simulink model "move_to_ball"  (R2020a)
settings: Solver=FixedStepDiscrete  StartTime=0.0  StopTime=inf  RelTol=1e-3
model workspace (MAT data in the model file):
  SL_ROS_VariableLengthArrays_MaxSizes.CommonInfo.ArrayTruncateAction = 'EmitWarning'
  SL_ROS_VariableLengthArrays_MaxSizes.MsgTypeMap = containers.Map
  SL_ROS_VariableLengthArrays_MaxSizes.MsgTypeMap.serialization.keys = {'sensor_msgs/Image'}
  SL_ROS_VariableLengthArrays_MaxSizes.MsgTypeMap.serialization.values{1}(1).PropertyName = 'Data'
  SL_ROS_VariableLengthArrays_MaxSizes.MsgTypeMap.serialization.values{1}(1).DataType = 'uint8'
  SL_ROS_VariableLengthArrays_MaxSizes.MsgTypeMap.serialization.values{1}(1).MaxLength = 3121200
  SL_ROS_VariableLengthArrays_MaxSizes.MsgTypeMap.serialization.values{1}(2).PropertyName = 'Encoding'
  SL_ROS_VariableLengthArrays_MaxSizes.MsgTypeMap.serialization.values{1}(2).DataType = 'uint8'
  SL_ROS_VariableLengthArrays_MaxSizes.MsgTypeMap.serialization.values{1}(2).MaxLength = 128
  SL_ROS_VariableLengthArrays_MaxSizes.MsgTypeMap.serialization.uniformity = 0
  SL_ROS_VariableLengthArrays_MaxSizes.MsgTypeMap.serialization.keyType = 'char'
  SL_ROS_VariableLengthArrays_MaxSizes.MsgTypeMap.serialization.valueType = 'any'
undefined symbols (not defined in the file): gray
libraries: robotlib x8
settings Model: Creator=shiva  LastModifiedBy=shiva
settings OptimizationCC: ZeroExternalMemoryAtStartup=off  ZeroInternalMemoryAtStartup=off
settings RTWCC: TargetLang=C++
settings GRTTargetCC: TargetLangStandard=C++03 (ISO)  MultiInstanceERTCode=on  CodeInterfacePackaging=C++ class

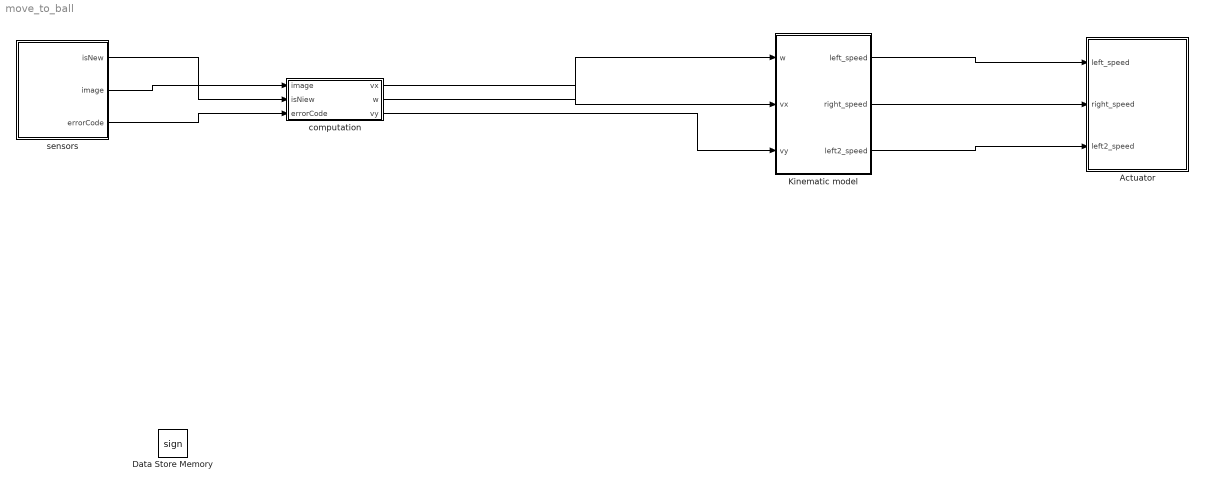
== system move_to_ball ==
  Actuator : Subsystem
  Data Store Memory : DataStoreMemory  DataStoreName=sign  ReadBeforeWriteMsg=warning  WriteAfterWriteMsg=warning  WriteAfterReadMsg=warning  ShowAdditionalParam=off
  Kinematic model : Subsystem
  computation : Subsystem
  sensors : Subsystem
  wires:
  Kinematic model/2(right_speed) -> Actuator/2(right_speed)
  Kinematic model/3(left2_speed) -> Actuator/3(left2_speed)
  Kinematic model/1(left_speed) -> Actuator/1(left_speed)
  sensors/1(isNew) -> computation/2(isNiew)
  sensors/2(image) -> computation/1(image)
  sensors/3(errorCode) -> computation/3(errorCode)
  computation/1(vx) -> Kinematic model/2(vx)
  computation/2(w) -> Kinematic model/1(w)
  computation/3(vy) -> Kinematic model/3(vy)

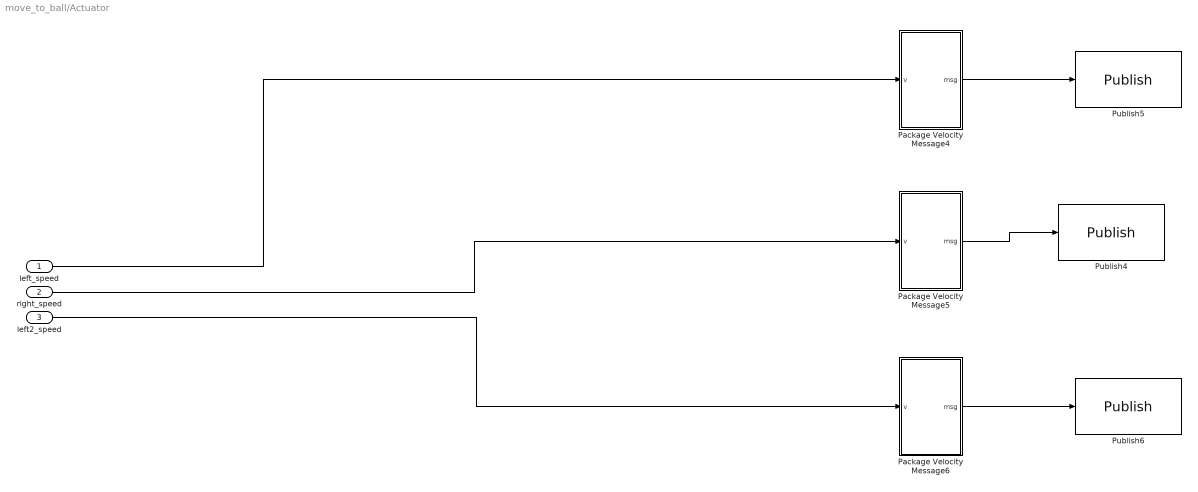
== system move_to_ball/Actuator ==
  left_speed : Inport
  right_speed : Inport  Port=2
  left2_speed : Inport  Port=3
  Package Velocity Message4 : Subsystem
  Package Velocity Message5 : Subsystem
  Package Velocity Message6 : Subsystem
  Publish4 : robotlib/Publish  topicSource=Select from ROS network  topic=/robot/right_joint_velocity_controller/command  messageType=std_msgs/Float64  messageQueueLength=1
  Publish5 : robotlib/Publish  topicSource=Select from ROS network  topic=/robot/left_joint_velocity_controller/command  messageType=std_msgs/Float64  messageQueueLength=1
  Publish6 : robotlib/Publish  topicSource=Select from ROS network  topic=/robot/left2_joint_velocity_controller/command  messageType=std_msgs/Float64  messageQueueLength=1
  wires:
  left_speed/1 -> Package Velocity Message4/1(v)
  Package Velocity Message6/1(msg) -> Publish6/1
  right_speed/1 -> Package Velocity Message5/1(v)
  Package Velocity Message4/1(msg) -> Publish5/1
  Package Velocity Message5/1(msg) -> Publish4/1
  left2_speed/1 -> Package Velocity Message6/1(v)

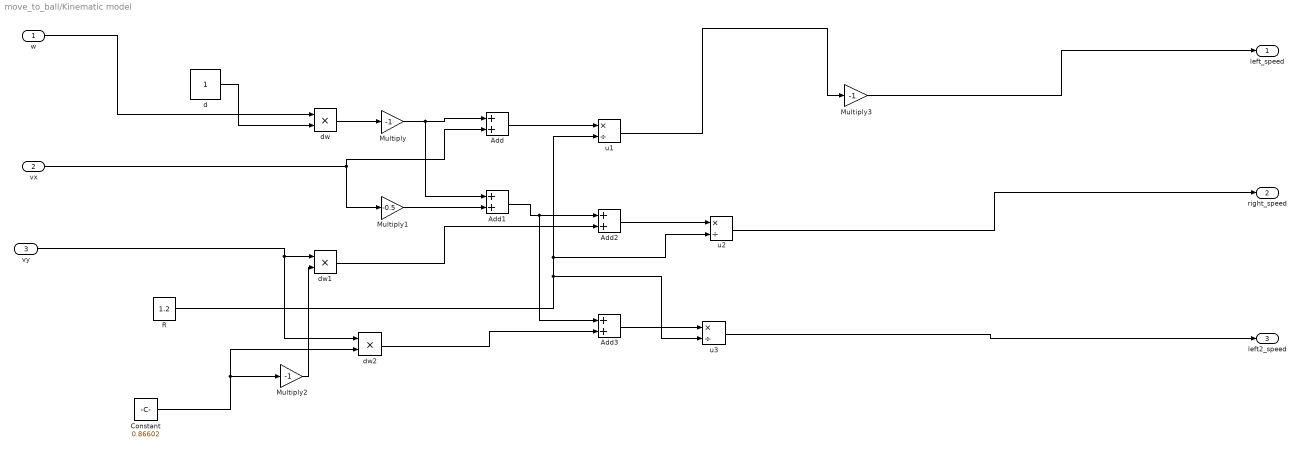
== system move_to_ball/Kinematic model ==
  w : Inport
  vx : Inport  Port=2
  vy : Inport  Port=3
  Add{,1..3} (4 alike) : Sum
  Constant : Constant  Value=0.86602
  Multiply : Gain  Gain=-1
  Multiply1 : Gain  Gain=-0.5
  Multiply2 : Gain  Gain=-1
  Multiply3 : Gain  Gain=-1
  R : Constant  Value=1.2
  d : Constant  VectorParams1D=off  SampleTime=-1
  dw : Product
  dw1 : Product
  dw2 : Product
  u1 : Product  Inputs=*/
  u2 : Product  Inputs=*/
  u3 : Product  Inputs=*/
  left_speed : Outport
  right_speed : Outport  Port=2
  left2_speed : Outport  Port=3
  wires:
  Multiply/1 -> Add1/1, Add/1
  Add/1 -> u1/1
  Multiply3/1 -> left_speed/1
  dw1/1 -> Add2/2
  w/1 -> dw/1
  Multiply2/1 -> dw1/2
  Add1/1 -> Add3/1, Add2/1
  Constant/1 -> dw2/2, Multiply2/1
  u3/1 -> left2_speed/1
  vy/1 -> dw2/1, dw1/1
  dw2/1 -> Add3/2
  d/1 -> dw/2
  u2/1 -> right_speed/1
  R/1 -> u3/2, u2/2, u1/2
  Add3/1 -> u3/1
  dw/1 -> Multiply/1
  vx/1 -> Add/2, Multiply1/1
  u1/1 -> Multiply3/1
  Add2/1 -> u2/1
  Multiply1/1 -> Add1/2

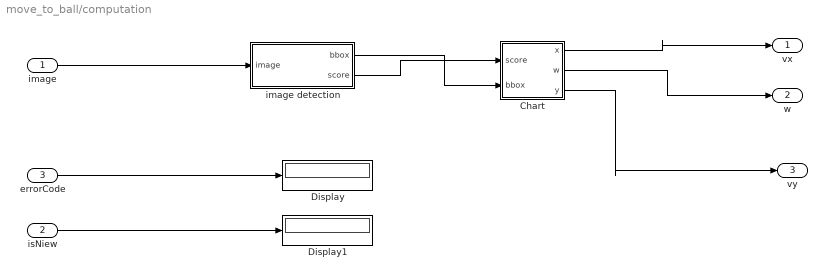
== system move_to_ball/computation ==
  image : Inport
  isNiew : Inport  Port=2
  errorCode : Inport  Port=3
  Chart : Stateflow chart  TreatAsAtomicUnit=on
  Display : Display
  Display1 : Display
  image detection : Subsystem
  vx : Outport
  w : Outport  Port=2
  vy : Outport  Port=3
  wires:
  image/1 -> image detection/1(image)
  errorCode/1 -> Display/1
  isNiew/1 -> Display1/1
  image detection/2(score) -> Chart/1(score)
  image detection/1(bbox) -> Chart/2(bbox)
  Chart/1(x) -> vx/1
  Chart/2(w) -> w/1
  Chart/3(y) -> vy/1

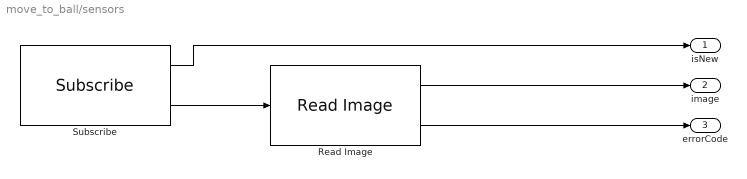
== system move_to_ball/sensors ==
  Read Image : robotlib/Read Image  MaximumImageSize=[1020, 1020]  ImageEncoding=rgb8  ShowAlphaOutput=off  ShowErrorCodeOutput=on  VariableSizeOutputs=off
      settings: SourceProductBaseCode=RR
  Subscribe : robotlib/Subscribe  topicSource=Select from ROS network  topic=/robot_sensor/camera/image_raw  messageType=sensor_msgs/Image  sampleTime=-1  messageQueueLength=1
  isNew : Outport
  image : Outport  Port=2
  errorCode : Outport  Port=3
  wires:
  Subscribe/2 -> Read Image/1
  Subscribe/1 -> isNew/1
  Read Image/1 -> image/1
  Read Image/2 -> errorCode/1

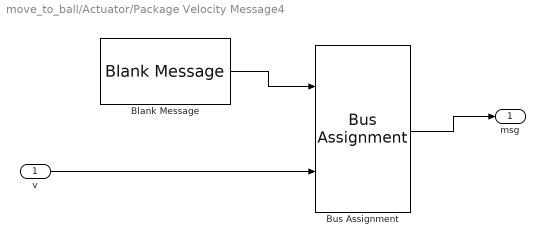
== system move_to_ball/Actuator/Package Velocity Message4 ==
  v : Inport
  Blank Message : robotlib/Blank Message  messageClass=Message  entityType=std_msgs/Float64  messageType=std_msgs/Float64  SampleTime=inf
  Bus Assignment : BusAssignment  AssignedSignals=Data
  msg : Outport  VectorParamsAs1DForOutWhenUnconnected=off
  wires:
  Blank Message/1 -> Bus Assignment/1
  Bus Assignment/1 -> msg/1
  v/1 -> Bus Assignment/2

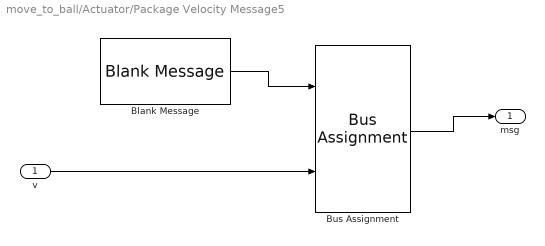
== system move_to_ball/Actuator/Package Velocity Message5 ==
  v : Inport
  Blank Message : robotlib/Blank Message  messageClass=Message  entityType=std_msgs/Float64  messageType=std_msgs/Float64  SampleTime=inf
  Bus Assignment : BusAssignment  AssignedSignals=Data
  msg : Outport  VectorParamsAs1DForOutWhenUnconnected=off
  wires:
  Blank Message/1 -> Bus Assignment/1
  Bus Assignment/1 -> msg/1
  v/1 -> Bus Assignment/2

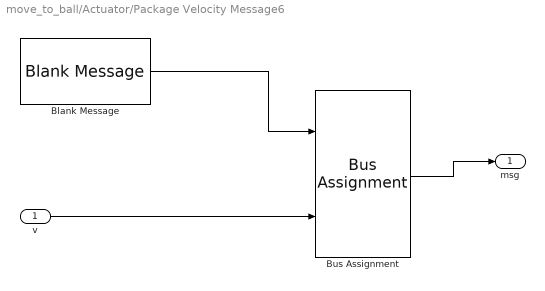
== system move_to_ball/Actuator/Package Velocity Message6 ==
  v : Inport
  Blank Message : robotlib/Blank Message  messageClass=Message  entityType=std_msgs/Float64  messageType=std_msgs/Float64  SampleTime=inf
  Bus Assignment : BusAssignment  AssignedSignals=Data
  msg : Outport  VectorParamsAs1DForOutWhenUnconnected=off
  wires:
  Blank Message/1 -> Bus Assignment/1
  Bus Assignment/1 -> msg/1
  v/1 -> Bus Assignment/2

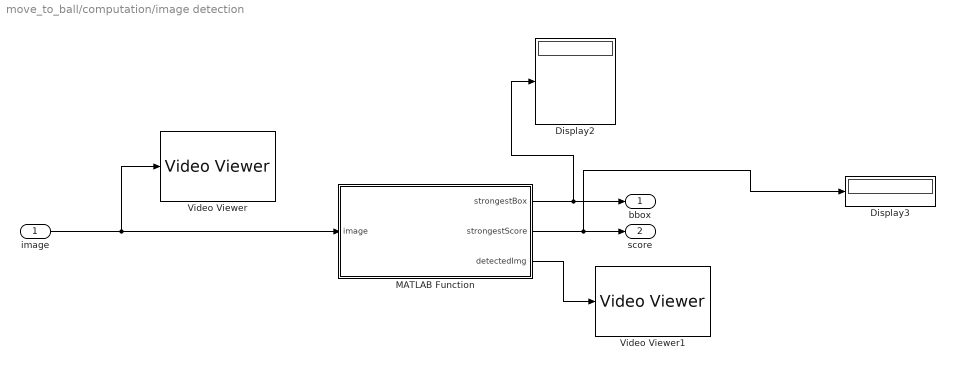
== system move_to_ball/computation/image detection ==
  image : Inport
  Display2 : Display
  Display3 : Display
  MATLAB Function : MATLAB Function  TreatAsAtomicUnit=on
  Video Viewer : VideoViewer  colormapValue=gray(256)  FigPos=[191 900 448 283]
  Video Viewer1 : VideoViewer  colormapValue=gray(256)  FigPos=[147 535 428 297]
  bbox : Outport
  score : Outport  Port=2
  wires:
  MATLAB Function/2(strongestScore) -> Display3/1, score/1
  MATLAB Function/1(strongestBox) -> Display2/1, bbox/1
  MATLAB Function/3(detectedImg) -> Video Viewer1/1
  image/1 -> Video Viewer/1, MATLAB Function/1(image)

== matlab function move_to_ball/computation/image detection/MATLAB Function ==
  data: image input; strongestBox output; strongestScore output; detectedImg output
function [strongestBox, strongestScore, detectedImg] = yolov2_detect(image)
strongestBox = zeros(1, 4);
strongestScore = 0;

imageResized = imresize(image,[224, 224]);
detectedImg = imageResized;
persistent yolov2Obj;

if isempty(yolov2Obj)
    yolov2Obj = coder.loadDeepLearningNetwork('yoloResNet50_det.mat');
end

[bboxes, scores] = yolov2Obj.detect(imageResized,'Threshold',0.1);

if(~isempty(bboxes))
    [strongestBox, strongestScore] = selectStrongestBbox(bboxes,scores,...
        'RatioType','Union',...
        'OverlapThreshold',0.5);
    strongestBox = strongestBox(1, :);
    strongestScore = double(strongestScore(1));
    
    detectedImg = insertObjectAnnotation(imageResized,'rectangle',...
        strongestBox,strongestScore, 'Color', [229, 0, 0]);
end
end

== stateflow chart move_to_ball/computation/Chart ==
  state no_ball
    w=0.8;
    x=0;
    y=0;
  state ball_in_middle
    if bbox(1) + bbox(3)/2 < 107
    w=1  * 0.3;;
    elseif bbox(1) + bbox(3)/2 > 117
    w=-1 * 0.3;
    end
    x=0;
    y = 0;
  state move_to_ball
    x=5;
    y=.86*5;
  (default) -> no_ball
  no_ball -> ball_in_middle : [score > 0.25]
  ball_in_middle -> move_to_ball : [bbox(1) + bbox(3)/2 > 107  && bbox(1) + bbox(3)/2 < 117]
  data: x output; w output; score input; bbox input; y output
